simulink model "fourinputslq_and_yaw_rate_control_sim"  (R2015a)
settings: Solver=ode45  StartTime=0.0  StopTime=15  FixedStep=ts  RelTol=1e-3
values from neighbouring files (symbols this model uses):
  A = eval(As)    [Three_torque_input.m]    (also in fourinputslq_and_yaw_rate_control.m; linearization.m)
  B = eval(Bs)    [Three_torque_input.m]    (also in fourinputslq_and_yaw_rate_control.m; linearization.m)
  Cs = [1 0 0 0 0 0; 0 1 0 0 0 0; 0 0 1 0 0 0;  0 0 0 1 0 0;0 0 0 0 1 0]    [Three_torque_input.m]    (also in fourinputslq_and_yaw_rate_control.m; linearization.m)
  Kr = -inv(Cc*inv(Aa-Bb*K)*Bb)    [Three_torque_input.m]    (also in fourinputslq_and_yaw_rate_control.m = -inv(Cc*inv(Aa-Bb*K)*Bb(:,2:4)); linearization.m = -inv(Cc*inv(Aa-Bb*Kk-eye(5))*Bb))
  Krd = -inv(Cc*inv(sysd.a-sysd.b*Kd-eye(5))*sysd.b(:,2:4))    [fourinputslq_and_yaw_rate_control.m]
  sysD = ss(A,B,eye(6),0,ts)    [fourinputslq_and_yaw_rate_control.m]
  ts = 1e-3    (= 0.001)    [fourinputslq_and_yaw_rate_control.m]
undefined symbols (not defined in the file or in its folder): K, Kd
settings Model: Creator=Jaby  LastModifiedBy=Jaby

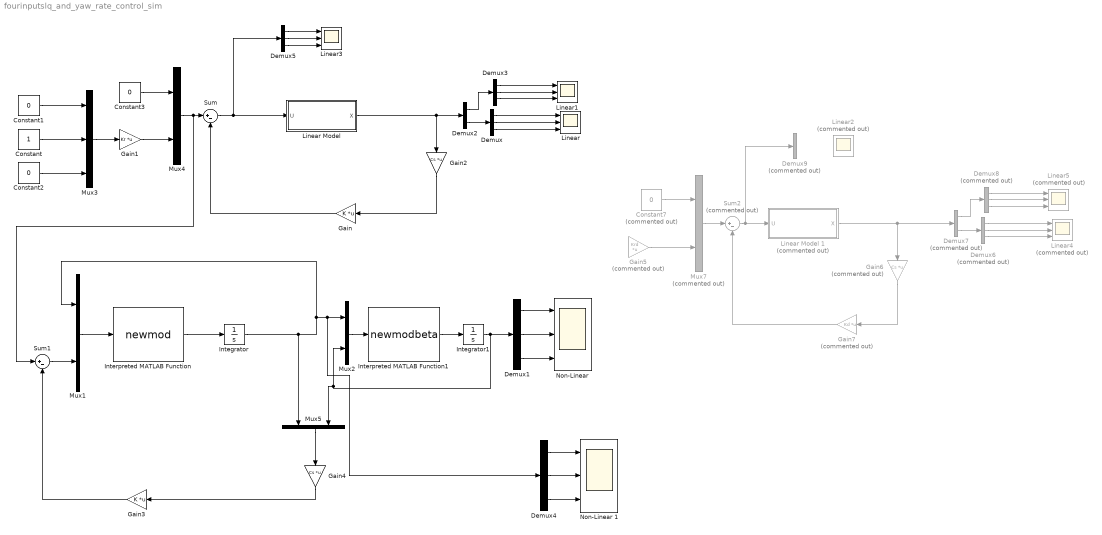
== system fourinputslq_and_yaw_rate_control_sim ==
  Constant : Constant  VectorParams1D=off
  Constant1 : Constant  Value=0  VectorParams1D=off
  Constant2 : Constant  Value=0  VectorParams1D=off
  Constant3 : Constant  Value=0  VectorParams1D=off
  Constant7 : Constant  Commented=on  Value=0  VectorParams1D=off
  Demux{,1,3..5} (5 alike) : Demux  Outputs=3
  Demux2 : Demux  Outputs=2
  Demux6 : Demux  Commented=on  Outputs=3
  Demux7 : Demux  Commented=on  Outputs=2
  Demux8 : Demux  Commented=on  Outputs=3
  Demux9 : Demux  Commented=on  Outputs=3
  Gain : Gain  Gain=K  Multiplication=Matrix(K*u)
  Gain1 : Gain  Gain=Kr  Multiplication=Matrix(K*u)
  Gain2 : Gain  Gain=Cs  Multiplication=Matrix(K*u)
  Gain3 : Gain  Gain=K  Multiplication=Matrix(K*u)
  Gain4 : Gain  Gain=Cs  Multiplication=Matrix(K*u)
  Gain5 : Gain  Commented=on  Gain=Krd  Multiplication=Matrix(K*u)
  Gain6 : Gain  Commented=on  Gain=Cs  Multiplication=Matrix(K*u)
  Gain7 : Gain  Commented=on  Gain=Kd  Multiplication=Matrix(K*u)
  Integrator : Integrator  InitialCondition=[0 0 0]'
  Integrator1 : Integrator  InitialCondition=[0 0 0]'
  Interpreted MATLAB Function : MATLABFcn  MATLABFcn=newmod  Output1D=off
  Interpreted MATLAB Function1 : MATLABFcn  MATLABFcn=newmodbeta  Output1D=off
  Linear : Scope  NumInputPorts=3
      settings: TimeRange=20  YMin=0.00274~-3.07e-14~8.3e-31  YMax=0.00278~-3.025e-14~8.43e-31
  "Linear Model " : Subsystem
  Linear Model 1 : Subsystem  Commented=on
  Linear1 : Scope  NumInputPorts=3
      settings: TimeRange=20  YMin=-0.5~-0.5~0  YMax=2.5~2.5~0.7000000000000001  SaveName=ScopeData2
  Linear2 : Scope  Commented=on  NumInputPorts=3
      settings: TimeRange=20  YMin=0.00274~-3.07e-14~8.3e-31  YMax=0.00278~-3.025e-14~8.43e-31  SaveName=ScopeData5
  Linear3 : Scope  NumInputPorts=3
      settings: TimeRange=20  YMin=0.00274~-3.07e-14~8.3e-31  YMax=0.00278~-3.025e-14~8.43e-31  SaveName=ScopeData4
  Linear4 : Scope  Commented=on  NumInputPorts=3
      settings: TimeRange=20  YMin=0.00274~-3.07e-14~8.3e-31  YMax=0.00278~-3.025e-14~8.43e-31  SaveName=ScopeData6
  Linear5 : Scope  Commented=on  NumInputPorts=3
      settings: TimeRange=20  YMin=-0.5~-0.5~0  YMax=2.5~2.5~0.7000000000000001  SaveName=ScopeData7
  Mux{1..2,4..5} (4 alike) : Mux  Inputs=2
  Mux3 : Mux  Inputs=3
  Mux7 : Mux  Commented=on  Inputs=2
  "Non-Linear " : Scope  NumInputPorts=3
      settings: YMin=-5~-5~-5  YMax=5~5~5
  Non-Linear 1 : Scope  NumInputPorts=3
      settings: YMin=-5~-5~-5  YMax=5~5~5  SaveName=ScopeData3
  Sum : Sum  Inputs=|+-
  Sum1 : Sum  Inputs=|+-
  Sum2 : Sum  Commented=on  Inputs=|+-
  wires:
  Demux/1 -> Linear/1
  Demux/2 -> Linear/2
  Demux/3 -> Linear/3
  Integrator/1 -> Mux5/1, Demux4/1, Mux2/1, Mux1/1
  Mux1/1 -> Interpreted MATLAB Function/1
  Interpreted MATLAB Function/1 -> Integrator/1
  Interpreted MATLAB Function1/1 -> Integrator1/1
  Demux1/2 -> "Non-Linear "/2
  Integrator1/1 -> Demux1/1, Mux5/2, Mux2/2
  Demux1/3 -> "Non-Linear "/3
  Demux1/1 -> "Non-Linear "/1
  Gain/1 -> Sum/2
  Demux2/2 -> Demux/1
  Mux3/1 -> Gain1/1
  Constant/1 -> Mux3/2
  Constant1/1 -> Mux3/1
  Demux3/1 -> Linear1/1
  Demux3/2 -> Linear1/2
  Demux3/3 -> Linear1/3
  Demux2/1 -> Demux3/1
  Constant2/1 -> Mux3/3
  "Linear Model "/1(X) -> Gain2/1, Demux2/1
  Mux4/1 -> Sum1/1, Sum/1
  Gain1/1 -> Mux4/2
  Constant3/1 -> Mux4/1
  Demux5/1 -> Linear3/1
  Demux5/2 -> Linear3/2
  Demux5/3 -> Linear3/3
  Sum/1 -> Demux5/1, "Linear Model "/1(U)
  Gain2/1 -> Gain/1
  Gain4/1 -> Gain3/1
  Gain3/1 -> Sum1/2
  Sum1/1 -> Mux1/2
  Mux5/1 -> Gain4/1
  Demux4/2 -> Non-Linear 1/2
  Mux2/1 -> Interpreted MATLAB Function1/1
  Demux4/3 -> Non-Linear 1/3
  Demux4/1 -> Non-Linear 1/1
  Gain7/1 -> Sum2/2
  Mux7/1 -> Sum2/1
  Gain5/1 -> Mux7/2
  Constant7/1 -> Mux7/1
  Sum2/1 -> Linear Model 1/1(U), Demux9/1
  Gain6/1 -> Gain7/1
  Demux6/1 -> Linear4/1
  Demux6/2 -> Linear4/2
  Demux6/3 -> Linear4/3
  Demux7/2 -> Demux6/1
  Demux8/1 -> Linear5/1
  Demux8/2 -> Linear5/2
  Demux8/3 -> Linear5/3
  Demux7/1 -> Demux8/1
  Linear Model 1/1(X) -> Demux7/1, Gain6/1

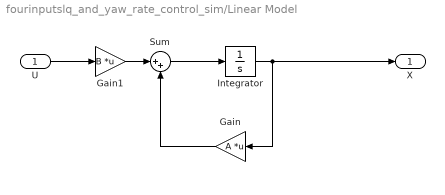
== system fourinputslq_and_yaw_rate_control_sim/Linear Model  ==
  U : Inport
  Gain : Gain  Gain=A  Multiplication=Matrix(K*u)
  Gain1 : Gain  Gain=B  Multiplication=Matrix(K*u)
  Integrator : Integrator
  Sum : Sum  Inputs=|++
  X : Outport
  wires:
  Integrator/1 -> X/1, Gain/1
  U/1 -> Gain1/1
  Gain1/1 -> Sum/1
  Sum/1 -> Integrator/1
  Gain/1 -> Sum/2

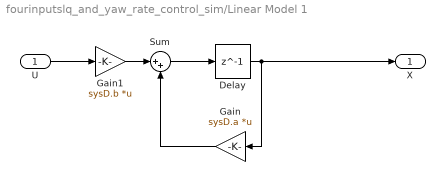
== system fourinputslq_and_yaw_rate_control_sim/Linear Model 1 ==
  U : Inport
  Delay : Delay  DelayLength=1  SampleTime=ts
  Gain : Gain  Gain=sysD.a  Multiplication=Matrix(K*u)
  Gain1 : Gain  Gain=sysD.b  Multiplication=Matrix(K*u)
  Sum : Sum  Inputs=|++
  X : Outport
  wires:
  Gain/1 -> Sum/2
  Sum/1 -> Delay/1
  Gain1/1 -> Sum/1
  U/1 -> Gain1/1
  Delay/1 -> X/1, Gain/1
